simulink model "SimBenchmark"  (R2025b)
settings: Solver=FixedStepAuto  StartTime=0.0  StopTime=50  FixedStep=Ts  RelTol=1e-3
values from neighbouring files (symbols this model uses):
  hiddenLayerSizeCtrl = 20    [Init.m]    (also in InitBenchmark.m)
  hiddenLayerSizeObsv = 5    [Init.m]    (also in InitBenchmark.m)
  p = 1    [Init.m]    (also in InitBenchmark.m; SimPlots.m; SimPlotsBenchmark.m; SimPlotsDiffq.m)
  q = 50    [InitBenchmark.m]    (also in Sat_qPlot.m = [2, 5, 11.5]; Sat_qPlotVertical.m = [2, 5, 11.5])
  rho = 2    [InitBenchmark.m]    (also in SimPlots.m = out.rho.signals.values; SimPlotsBenchmark.m; SimPlotsV1.m = out.rho.signals.values)
  u_max = 5    [Init.m]    (also in InitBenchmark.m = 2; SimPlots.m = 2; SimPlotsBenchmark.m = 1.5; SimPlotsDiffq.m = 1)
  u_min = - 5    (= -5)    [Init.m]    (also in InitBenchmark.m = -2; SimPlots.m = -2; SimPlotsBenchmark.m = -1.5; SimPlotsDiffq.m = -1)
  Vctrl0 = 0.1 * randn(hiddenLayerSizeCtrl, inputLayerSizeCtrl)    [Init.m]    (also in InitBenchmark.m)
  Vobsv0 = 0.1 * randn(hiddenLayerSizeObsv, inputLayerSizeObsv)    [Init.m]    (also in InitBenchmark.m)
  Wctrl0 = 0.1 * randn(outputLayerSizeCtrl, hiddenLayerSizeCtrl)    [Init.m]    (also in InitBenchmark.m)
  Wobsv0 = 0.1 * randn(outputLayerSizeObsv, hiddenLayerSizeObsv)    [Init.m]    (also in InitBenchmark.m)
  x_hat0 = [0.9; 0]    [Init.m]    (also in InitBenchmark.m = [-0.2; 0])
  zeta0 = [0.5; 0; 0.5]    [InitBenchmark.m]
settings Model: Creator=Asus  LastModifiedBy=Asus

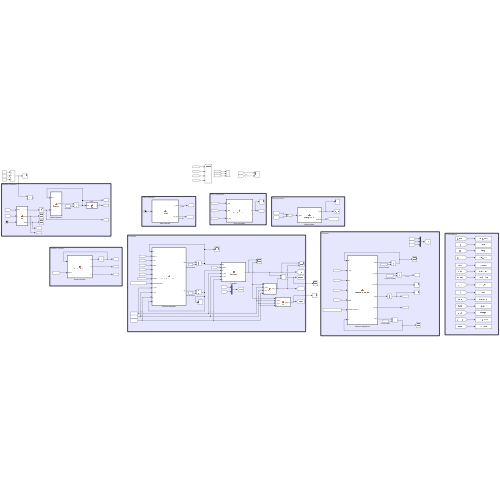
[thumbnail: Simulink's stored preview of the top-level diagram]
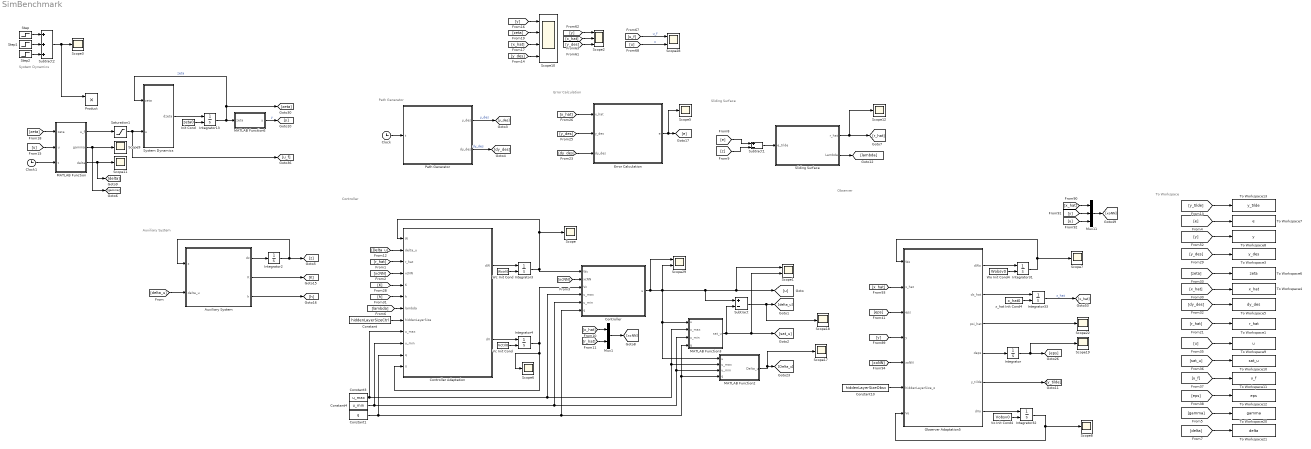
== system SimBenchmark ==
  note: Path Generator
  note: Auxiliary System
  note: Controller
  note: Sliding Surface
  note: Error Calculation
  note: Observer
  note: System Dynamics
  note: To Workspace
  Auxiliary System : MATLAB Function  TreatAsAtomicUnit=on
  Clock : Clock
  Clock1 : Clock
  Constant : Constant  Value=hiddenLayerSizeCtrl
  Constant1 : Constant  Value=q
  Constant10 : Constant  Value=hiddenLayerSizeObsv
  Constant3 : Constant  Value=u_max
  Constant4 : Constant  Value=u_min
  Controller : MATLAB Function  TreatAsAtomicUnit=on
  Controller Adaptation : MATLAB Function  TreatAsAtomicUnit=on
  Error Calculation : MATLAB Function  TreatAsAtomicUnit=on
  Init Cond : Constant  Value=zeta0
  Integrator : Integrator  InitialCondition=5 * ones(p, 1)
  Integrator{3..4,13,31..33} (6 alike) : Integrator  InitialConditionSource=external  InitialCondition=[0.5; 0.5]
  Integrator2 : Integrator  InitialCondition=zeros(rho, 1)
  MATLAB Function : MATLAB Function  TreatAsAtomicUnit=on
  MATLAB Function2 : MATLAB Function  TreatAsAtomicUnit=on
  MATLAB Function3 : MATLAB Function  TreatAsAtomicUnit=on
  MATLAB Function6 : MATLAB Function  TreatAsAtomicUnit=on
  Mux1 : Mux  Inputs=2
  Mux11 : Mux  Inputs=3
  Observer Adaptation5 : MATLAB Function  TreatAsAtomicUnit=on
  Path Generator : MATLAB Function  TreatAsAtomicUnit=on
  Product : Product
  Saturation1 : Saturate  UpperLimit=u_max  LowerLimit=u_min
  Scope{,3,5..9,11..12,17..19,22} (13 alike) : Scope
      Scope settings: ActiveDisplayYMinimum=-0.87201084140231888  ActiveDisplayYMaximum=1.1571514611092091
      Scope11 settings: ActiveDisplayYMinimum=-1  ActiveDisplayYMaximum=1  DataLoggingVariableName=ScopeData6
      Scope12 settings: ActiveDisplayYMinimum=-11.020649415601135  ActiveDisplayYMaximum=28.929403949894713  DataLoggingVariableName=ScopeData7
      Scope17 settings: ActiveDisplayYMinimum=-0.12499999999999997  ActiveDisplayYMaximum=1.125  DataLoggingVariableName=ScopeData17
      Scope18 settings: ActiveDisplayYMinimum=-1  ActiveDisplayYMaximum=1  DataLoggingVariableName=ScopeData20
      Scope19 settings: ActiveDisplayYMinimum=-3.2712431921817543E+56  ActiveDisplayYMaximum=7.3775862851276354E+57  DataLoggingVariableName=ScopeData15
      Scope22 settings: ActiveDisplayYMinimum=-0.7647026863167814  ActiveDisplayYMaximum=1.4700092233149542  DataLoggingVariableName=ScopeData18
      Scope3 settings: ActiveDisplayYMinimum=-1  ActiveDisplayYMaximum=1  DataLoggingVariableName=ScopeData4
      Scope5 settings: ActiveDisplayYMinimum=-0.549764200239591  ActiveDisplayYMaximum=0.44787780215631889
      Scope6 settings: ActiveDisplayYMinimum=-0.75292691508642251  ActiveDisplayYMaximum=0.86809325502056134  DataLoggingVariableName=ScopeData2
      Scope7 settings: ActiveDisplayYMinimum=-0.12846291127553625  ActiveDisplayYMaximum=0.10453389195897768  DataLoggingVariableName=ScopeData9
      Scope8 settings: ActiveDisplayYMinimum=-2.9041783435528368  ActiveDisplayYMaximum=2.5556532442981439  DataLoggingVariableName=ScopeData10
      Scope9 settings: ActiveDisplayYMinimum=0.66977640233126912  ActiveDisplayYMaximum=1.0366915108520809  DataLoggingVariableName=ScopeData5
  Scope1 : Scope  NumInputPorts=2
      settings: ActiveDisplayYMinimum=-3.7470635666671717  ActiveDisplayYMaximum=3.7485971330756858  DataLoggingVariableName=ScopeData3
  Scope10 : Scope  NumInputPorts=4
      settings: ActiveDisplayYMinimum=-1.7685834132779761  ActiveDisplayYMaximum=1.2578380503264766  DataLoggingVariableName=ScopeData11
  Scope2 : Scope  NumInputPorts=3
      settings: ActiveDisplayYMinimum=-0.8810106133872696  ActiveDisplayYMaximum=0.94290676291795084
  Scope28 : Scope  NumInputPorts=2
      settings: ActiveDisplayYMinimum=-2.4999703880393493  ActiveDisplayYMaximum=2.4997334923541432  DataLoggingVariableName=ScopeData24
  Scope29 : Scope  NumInputPorts=2
      settings: ActiveDisplayYMinimum=-6.1765297124862251  ActiveDisplayYMaximum=2.6873317974154434  DataLoggingVariableName=ScopeData28
  Sliding Surface : MATLAB Function  TreatAsAtomicUnit=on
  Step : Step  Time=0  SampleTime=0
  Step1 : Step  Time=10  After=-0.25  SampleTime=0
  Step2 : Step  Time=20  After=0.25  SampleTime=0
  Subtract : Sum  Inputs=+-
  Subtract1 : Sum  Inputs=+-
  Subtract2 : Sum  Inputs=+++
  System Dynamics : MATLAB Function  TreatAsAtomicUnit=on
  To Workspace1 : ToWorkspace  VariableName=r_hat  SaveFormat=Structure  SampleTime=-1
      settings: Save2DSignal=2-D array (concatenate along first dimension)
  To Workspace10 : ToWorkspace  VariableName=sat_u  SaveFormat=Structure  SampleTime=-1
      settings: Save2DSignal=2-D array (concatenate along first dimension)
  To Workspace11 : ToWorkspace  VariableName=u_f  SaveFormat=Structure  SampleTime=-1
      settings: Save2DSignal=2-D array (concatenate along first dimension)
  To Workspace12 : ToWorkspace  VariableName=eps  SaveFormat=Structure  SampleTime=-1
      settings: Save2DSignal=2-D array (concatenate along first dimension)
  To Workspace13 : ToWorkspace  VariableName=y_tilde  SaveFormat=Structure  SampleTime=-1
      settings: Save2DSignal=2-D array (concatenate along first dimension)
  To Workspace20 : ToWorkspace  VariableName=gamma  SaveFormat=Structure  SampleTime=-1
      settings: Save2DSignal=2-D array (concatenate along first dimension)
  To Workspace21 : ToWorkspace  VariableName=delta  SaveFormat=Structure  SampleTime=-1
      settings: Save2DSignal=2-D array (concatenate along first dimension)
  To Workspace3 : ToWorkspace  VariableName=y_des  SaveFormat=Structure  SampleTime=-1
      settings: Save2DSignal=2-D array (concatenate along first dimension)
  To Workspace4 : ToWorkspace  VariableName=x_hat  SaveFormat=Structure  SampleTime=-1
      settings: Save2DSignal=2-D array (concatenate along first dimension)
  To Workspace5 : ToWorkspace  VariableName=dy_des  SaveFormat=Structure  SampleTime=-1
      settings: Save2DSignal=2-D array (concatenate along first dimension)
  To Workspace6 : ToWorkspace  VariableName=zeta  SaveFormat=Structure  SampleTime=-1
      settings: Save2DSignal=2-D array (concatenate along first dimension)
  To Workspace7 : ToWorkspace  VariableName=e  SaveFormat=Structure  SampleTime=-1
      settings: Save2DSignal=2-D array (concatenate along first dimension)
  To Workspace8 : ToWorkspace  VariableName=y  SaveFormat=Structure  SampleTime=-1
      settings: Save2DSignal=2-D array (concatenate along first dimension)
  To Workspace9 : ToWorkspace  VariableName=u  SaveFormat=Structure  SampleTime=-1
      settings: Save2DSignal=2-D array (concatenate along first dimension)
  Vc Init Cond : Constant  Value=Vctrl0
  Vo Init Cond4 : Constant  Value=Vobsv0
  Wc Init Cond : Constant  Value=Wctrl0
  Wo Init Cond4 : Constant  Value=Wobsv0
  x_hat Init Cond4 : Constant  Value=x_hat0
  wires:
  Clock/1 -> Path Generator/1(t)
  Auxiliary System/1(dz) -> Integrator2/1
  Integrator2/1 -> [z], Auxiliary System/1(z)
  Wc Init Cond/1 -> Integrator3/2
  Controller Adaptation/1(dW) -> Integrator3/1
  Integrator3/1 -> Scope/1, Controller Adaptation/1(W), Controller/1(Wc)
  Controller Adaptation/2(dV) -> Integrator4/1
  Vc Init Cond/1 -> Integrator4/2
  Integrator4/1 -> Controller/3(Vc), Controller Adaptation/12(V), Scope6/1
  [r_hat] -> Controller Adaptation/3(r_hat)
  [xcNN] -> Controller Adaptation/4(xcNN)
  [xcNN] -> Controller/2(xcNN)
  Mux1/1 -> [xcNN]
  [Delta_u] -> Controller Adaptation/2(delta_u)
  Constant/1 -> Controller Adaptation/8(hiddenLayerSize)
  Sliding Surface/1(r_hat) -> Scope12/1, [r_hat]
  Path Generator/2(dy_des) -> [dy_des]  "dy_des"
  Path Generator/1(y_des) -> [y_des]  "y_des"
  [lambda] -> Controller Adaptation/7(lambda)
  Sliding Surface/2(Lambda) -> [lambda]
  [dy_des] -> Error Calculation/3(dy_des)
  [x_hat] -> Mux1/1
  [delta_u] -> Auxiliary System/2(delta_u)
  Subtract/1 -> Scope18/1, [delta_u]
  Observer Adaptation5/2(dx_hat) -> Integrator33/1
  Observer Adaptation5/6(dVo) -> Integrator32/1
  Mux11/1 -> [xoNN]
  [xoNN] -> Observer Adaptation5/5(xoNN)
  Integrator32/1 -> Observer Adaptation5/7(Vo), Scope8/1
  [u] -> Mux11/3
  [y] -> Observer Adaptation5/4(y)
  Wo Init Cond4/1 -> Integrator31/2
  Constant10/1 -> Observer Adaptation5/6(hiddenLayerSize_o)
  [x_hat] -> Observer Adaptation5/2(x_hat)
  Integrator31/1 -> Scope7/1, Observer Adaptation5/1(Wo)
  x_hat Init Cond4/1 -> Integrator33/2
  [x_hat] -> Mux11/1
  Vo Init Cond4/1 -> Integrator32/2
  [y] -> Mux11/2
  [x_hat] -> Error Calculation/1(x_hat)
  Integrator13/1 -> System Dynamics/1(zeta), [zeta], MATLAB Function6/1(zeta)  "zeta"
  System Dynamics/1(dzeta) -> Integrator13/1
  Init Cond/1 -> Integrator13/2
  Observer Adaptation5/1(dWo) -> Integrator31/1
  MATLAB Function2/1(Delta_u) -> Scope17/1, [Delta_u]
  Constant3/1 -> Controller Adaptation/9(u_max), Controller/4(u_max), MATLAB Function3/2(u_max), MATLAB Function2/2(u_max)
  Constant4/1 -> Controller Adaptation/10(u_min), Controller/5(u_min), MATLAB Function2/3(u_min), MATLAB Function3/3(u_min)
  Integrator33/1 -> [x_hat]  "x_hat"
  Observer Adaptation5/4(deps) -> Integrator/1
  Integrator/1 -> Scope19/1, [eps]
  [eps] -> Observer Adaptation5/3(eps)
  Observer Adaptation5/3(psi_hat) -> Scope22/1
  [e] -> Subtract1/1
  Subtract1/1 -> Sliding Surface/1(e_tilde)
  [z] -> Subtract1/2
  [y] -> Scope2/1
  Saturation1/1 -> System Dynamics/2(u), [u_f]
  [u_f] -> Scope28/1  "u_f"
  [u] -> Scope28/2  "u"
  Clock1/1 -> MATLAB Function/3(t)
  [u] -> MATLAB Function/2(u)
  [zeta] -> MATLAB Function/1(zeta)
  MATLAB Function/2(gamma) -> Scope9/1, [gamma]
  MATLAB Function/3(delta) -> [delta], Scope11/1
  [K] -> Controller Adaptation/5(K)
  [h] -> Controller Adaptation/6(h)
  Auxiliary System/2(K) -> [K]
  Auxiliary System/3(h) -> [h]
  [x_hat] -> Scope2/2
  [y_des] -> Scope2/3
  [dy_des] -> To Workspace5/1
  [y_des] -> To Workspace3/1
  [eps] -> To Workspace12/1
  [sat_u] -> To Workspace10/1
  [r_hat] -> To Workspace1/1
  [y] -> To Workspace8/1
  [u] -> To Workspace9/1
  [u_f] -> To Workspace11/1
  [zeta] -> To Workspace6/1
  [x_hat] -> To Workspace4/1
  [gamma] -> To Workspace20/1
  [delta] -> To Workspace21/1
  [e] -> To Workspace7/1
  Observer Adaptation5/5(y_tilde) -> [y_tilde]
  [y_tilde] -> To Workspace13/1
  MATLAB Function3/1(sat_u) -> Subtract/2, Scope1/2, [sat_u]
  MATLAB Function6/1(y) -> [y]  "y"
  [y] -> Scope10/1
  [x_hat] -> Scope10/3
  [y_des] -> Scope10/4
  [r_hat] -> Mux1/2
  Controller/1(u) -> Scope1/1, [u], Subtract/1, Scope29/2, MATLAB Function3/1(u), MATLAB Function2/1(u), Scope29/1
  Error Calculation/1(e) -> Scope5/1, [e]
  [y_des] -> Error Calculation/2(y_des)
  [zeta] -> Scope10/2
  Constant1/1 -> Controller Adaptation/11(q), Controller/6(q), MATLAB Function2/4(q), MATLAB Function3/4(q)
  Step/1 -> Subtract2/1
  Step1/1 -> Subtract2/2
  Step2/1 -> Subtract2/3
  Subtract2/1 -> Product/1, Scope3/1
  MATLAB Function/1(u_f) -> Saturation1/1

== matlab function SimBenchmark/Controller ==
  data: u output; Wc input; xcNN input; Vc input; u_max input; u_min input; q input
function u = Controller(Wc, xcNN, Vc, u_max, u_min, q)

    sat_q = @(u) (u_max+u_min)/2 + (u - (u_max+u_min)/2) / (1 + abs((u - (u_max+u_min)/2)/((u_max-u_min)/2))^q)^(1/q);

    Sigma = @(z) (-1 + 2 ./ (1 + exp(-2 * z)));
    u = - sat_q(Wc' * Sigma(Vc * xcNN));
    
end

== matlab function SimBenchmark/Controller Adaptation ==
  data: dW output; dV output; W input; delta_u input; r_hat input; xcNN input; K input; h input; lambda input; hiddenLayerSize input; u_max input; u_min input; q input; V input
function [dW, dV] = ControllerAdaptation(W, delta_u, r_hat, xcNN, K, h, lambda, hiddenLayerSize, u_max, u_min, q, V)
    
    Sigma = @(z) (-1 + 2 ./ (1 + exp(-2 * z)));
    Sigma_c  = Sigma(V * xcNN);

    l = 2;

    A = [0, 1; 0, 0];
    B = [0; 1];

    Ac = A - B * ([lambda', 1] * l + [0, lambda']);

    eta   = 10 * [0.1, 0.1];
    gamma = [0.0005, 0.0005];

    PI_c      = diag(Sigma_c.^2);
    PI_lambda = [lambda', 1];

    Psi_1c = (1 + abs((W' * Sigma(V * xcNN) - (u_max+u_min)/2)/((u_max-u_min)/2))^q)^(-(q+1)/q);
    
    dW = eta(1) * (r_hat' * PI_lambda * (-Ac^(-1) * B + K^(-1) * h * diag(delta_u)) * Psi_1c)' * Sigma_c' - gamma(1) * norm(r_hat) * W';
    dV = eta(2) * (r_hat' * PI_lambda * Psi_1c * (-Ac^(-1) * B + K^(-1) * h * diag(delta_u)) * W' * (eye(hiddenLayerSize) - PI_c))' * xcNN' - gamma(2) * norm(r_hat) * V;

end

== matlab function SimBenchmark/Sliding Surface ==
  data: e_tilde input; r_hat output; Lambda output
function [r_hat, Lambda] = SlidingSurface(e_tilde)

    Lambda = 8;

    r_hat = [Lambda, 1] * e_tilde;

end

== matlab function SimBenchmark/Error Calculation ==
  data: e output; x_hat input; y_des input; dy_des input
function e = ErrorCalculation(x_hat, y_des, dy_des)

    y_bar_des = [y_des; dy_des];
    e = x_hat - y_bar_des;
    
end

== matlab function SimBenchmark/MATLAB Function2 ==
  data: u input; Delta_u output; u_max input; u_min input; q input
function Delta_u = fcn(u, u_max, u_min, q)

    % if u > u_max
    %     Delta_u   = 1;
    % elseif u < u_min
    %     Delta_u   = 1;
    % else
    %     Delta_u   = 0;
    % end

    Delta_u = 1 - (1 + abs((u - (u_max+u_min)/2)/((u_max-u_min)/2))^q)^(-(q+1)/q);

end

== matlab function SimBenchmark/MATLAB Function3 ==
  data: u input; sat_u output; u_max input; u_min input; q input
function sat_u = fcn(u, u_max, u_min, q)

    sat_u = (u_max+u_min)/2 + (u - (u_max+u_min)/2) / (1 + abs((u - (u_max+u_min)/2)/((u_max-u_min)/2))^q)^(1/q);

end

== matlab function SimBenchmark/MATLAB Function6 ==
  data: y output; zeta input
function y = fcn(zeta)

    y  = 0.3*zeta(1)^3 - 0.5*zeta(1)^2 + zeta(1);

end

== matlab function SimBenchmark/System Dynamics ==
  data: zeta input; dzeta output; u input
function dzeta = Dynamics(zeta, u)

    dzeta    = zeros(3, 1);
    dzeta(1) = zeta(2) + sin(zeta(1));
    dzeta(2) = zeta(1) + zeta(3) + zeta(2)^2 + tanh(zeta(1)) + log(1 + zeta(1)^2 + zeta(3)^2) + (2 + cos(zeta(1))) * u + 0.1 * u^3;
    dzeta(3) = - zeta(3) - zeta(3)^3 + sin(zeta(1)*zeta(3));


    % A = [0, 1; 6, 5];
    % B = [0, 1]';
    % 
    % dzeta(1:2) = A * zeta(1:2) + B * u;
    % dzeta(3) = - zeta(3);

end

== matlab function SimBenchmark/Observer Adaptation5 ==
  data: dWo output; dx_hat output; psi_hat output; deps output; y_tilde output; dVo output; Wo input; x_hat input; eps input; y input; xoNN input; hiddenLayerSize_o input; Vo input
function [dWo, dx_hat, psi_hat, deps, y_tilde, dVo] = ObserverAdaptation(Wo, x_hat, eps, y, xoNN, hiddenLayerSize_o, Vo)

    Sigma = @(z) (-1 + 2 ./ (1 + exp(-2 * z)));
    Sigma_o = Sigma(Vo * xoNN);

    A = [0, 1; 0, 0];
    B = [0; 1];
    C = [1; 0];
    
    y_hat   = C' * x_hat;
    y_tilde = y - y_hat;

    alpha  = [1, 2];
    lambda = 0.01;
    kappa  = 50 ./ lambda;

    psi_hat = Wo' * Sigma_o;

    if norm(y_tilde) > lambda
        % deps = kappa * norm(y_tilde) + (eps - 10) * norm(y_tilde);
        % deps = - 10 * (eps - 50) * norm(y_tilde);
        deps = kappa * norm(y_tilde);
    else
        % deps = - 100 * lambda * eps;
        deps = 0;
    end

    % deps = kappa * norm(y_tilde) - 10 * norm(psi_hat);
    % deps = 50 * norm(y_tilde) / (1 + 10 * norm(Wo));
    % deps = 50 * norm(y_tilde) * exp(-3 * norm(Wo));

    % deps = kappa * norm(y_tilde) * tanh(norm(y_tilde) / 0.1) - 0.2 * kappa * (eps - 1);

    % deps = 0;

    rho   = 2;
    H     = zeros(rho, 1);
    for i = 1:rho
        H(i, 1) = alpha(1, i) * eps^i;
    end
    
    Ao   = A  - H*C';

    dx_hat  = A * x_hat + B * psi_hat + H * y_tilde;

    eta_o   = 0.20 * [10, 10];
    % eta_o   = 10 * 1/eps * [10, 10];
    gamma_o = 0.010 * [0.01, 0.01];

    PI_o = diag(Sigma_o.^2);

    dWo = - eta_o(1) * (y_tilde' * C' * Ao^(-1) * B)' * Sigma_o' - gamma_o(1) * norm(y_tilde) * Wo';
    dVo = - eta_o(2) * (y_tilde' * C' * Ao^(-1) * B * Wo' * (eye(hiddenLayerSize_o) - PI_o))' * xoNN' - gamma_o(2) * norm(y_tilde) * Vo;


    % Psi_1o = (Sigma_o * (C' * Ao^(-1) * B)')';
    % Psi_2o = (xoNN * C' * Ao^(-1) * B * Wo' * (eye(hiddenLayerSize_o) - PI_o))';
    % 
    % dWo = - eta_o(1) * (Psi_1o / (1 + Psi_1o' * Psi_1o)) * y_tilde - gamma_o(1) * norm(y_tilde) * Wo';
    % dVo = - eta_o(2) * (Psi_2o / (1 + Psi_2o' * Psi_2o)) * y_tilde - gamma_o(2) * norm(y_tilde) * Vo;


     

end

== matlab function SimBenchmark/Auxiliary System ==
  data: z input; dz output; delta_u input; K output; h output
function [dz, K, h] = AuxiliarySystem(z, delta_u)
    
    K = 5  * diag([-1, -1]);
    h = 0.05 * [-1; -1];

    dz = K * z + h .* delta_u;
    
end

== matlab function SimBenchmark/MATLAB Function ==
  data: zeta input; u input; u_f output; t input; gamma output; delta output
function [u_f, gamma, delta] = fcn(zeta, u, t)

    a     = 0.8;
    b     = 0.05;
    gamma   = a + (1-a) * exp(-0.2 * t) + b * sin(10 * t) + b * cos(10 * t + sin(t) + pi/3) - b/2;
    % f = 0;
    % if t > 20 && t<30
    f = 0.2 * sin(t) - 0.2 * cos(2*(t))^2;
    % end
    delta = (0.2 * cos(pi/3-tanh(zeta(1))^2) * sin(zeta(1)) + f);
    u_f   = gamma .* u + delta;

    % u_f = u;

end

== matlab function SimBenchmark/Path Generator ==
  data: t input; y_des output; dy_des output
function [y_des, dy_des] = PathGen(t)
    
    y_des   =   0.5 * cos(0.7 * t + pi/3) + 0.2 * sin(1.8 * t);
    dy_des  = - 0.5 * 0.7 * sin(0.7 * t + pi/3) + 0.2 * 1.8 * cos(1.8 * t);
    
end
